simulink model "linear_sys"  (R2021b)
settings: Solver=VariableStepAuto  StartTime=0.0  StopTime=5  RelTol=1e-3
values from neighbouring files (symbols this model uses):
  beta = 15    [run_6dof.m]
  Cldp = U(21)    [totalfm.m]
  Cmdq = U(19)    [totalfm.m]
  Cmq = U(18)    [totalfm.m]
  d = 265/1000    (= 0.265)    [run_6dof.m]
  damp = 0.9    [run_6dof.m]
  g = 9.81    [run_6dof.m]
  K1 = 4.3    [run_6dof.m]
  K2 = 0.2    [run_6dof.m]
  K3 = 0.3    [run_6dof.m]
  KP = 2    [run_6dof.m]
  m = fixed_mass+N2O_mass+Fuel_mass    [CG_CPcal.m]    (also in Rocket_property.m = 168.84; totalfm.m = U(28))
  qbar = U(10)    [totalfm.m]
  S = 1/4*pi*d^2    (= 0.0551545860246)    [run_6dof.m]
  theta = acos(1-2*X/lnose)    [plotDatcomAeroGeometry_221130.m]
  tou1 = 5/wg    (= 2.5)    [run_6dof.m]
  tou2 = 1/wm*sqrt(1/afa)    [run_6dof.m]
  V = U(31)    [totalfm.m]
  wn = BW/sqrt(1-2*damp^2+sqrt(2-4*damp^2+4*damp^4))    [run_6dof.m]
undefined symbols (not defined in the file or in its folder): alpha, CAN_TRANS_FREQ, Clp, Cma, Cna, Cnq, IMU_SAMP_FREQ, Ix, Iy, n, o
libraries: simulink_extras x9, simulink x3, dspsigops x3, slctrlblks x2
settings Model: Creator=310611102  LastModifiedBy=310611102

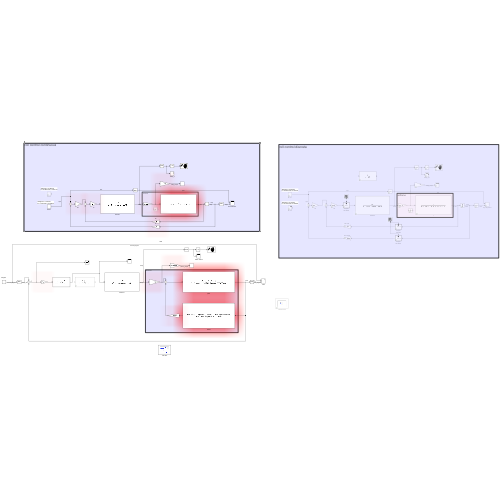
[thumbnail: Simulink's stored preview of the top-level diagram]
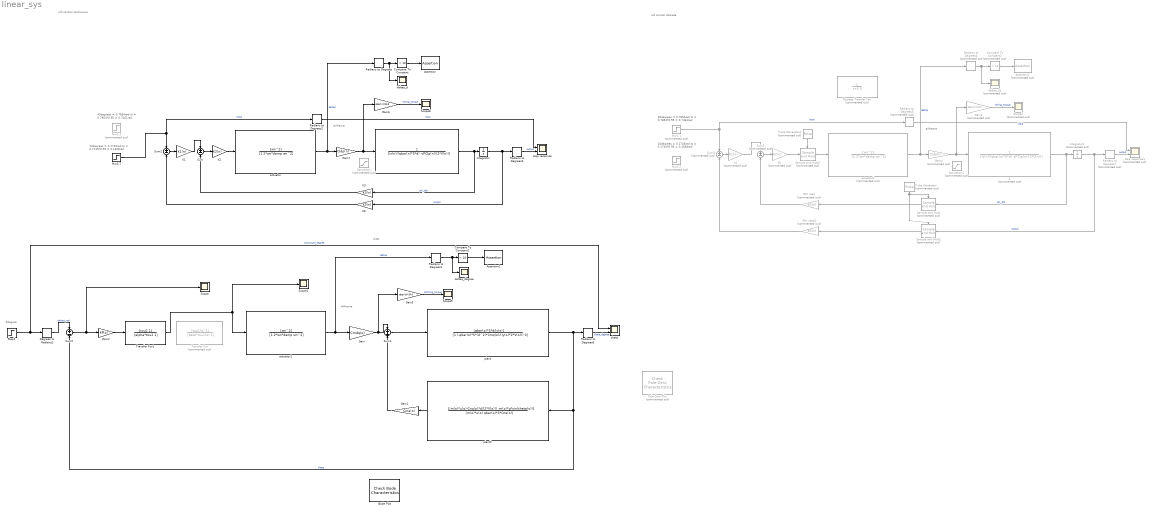
== system linear_sys ==
  note: roll control continuous
  note: 5degree
  note: airframe
  note: Airframe
  note: 45degrees = 0.7854rad
      | ts = 0.7854*0.95 = 0.7461rad
  note: C2D
  note: 10degrees = 0.1745rad
      | ts = 0.1745*0.95 = 0.1658rad
  note: airframe
  note: 45degrees = 0.7854rad
      | ts = 0.7854*0.95 = 0.7461rad
  note: 10degrees = 0.1745rad
      | ts = 0.1745*0.95 = 0.1658rad
  note: roll control discrete
  " " : TransferFcn  Numerator=1  Denominator=[Ix(n)/(qbar(n)*S*d) -d*Clp(n)/(2*V(n))]
  " 1" : TransferFcn  Commented=on  Numerator=1  Denominator=[Ix(n)/(qbar(n)*S*d) -d*Clp(n)/(2*V(n))]
  Assertion : Assertion  Enabled=off  AssertionFailFcn="error(\"large deflection angle\")"  StopWhenAssertionFail=off
  Assertion1 : Assertion  Enabled=off  AssertionFailFcn="error(\"large deflection angle\")"  StopWhenAssertionFail=off
  Assertion2 : Assertion  Commented=on  Enabled=off  AssertionFailFcn="error(\"large deflection angle\")"  StopWhenAssertionFail=off
  Bode Plot : slctrlblks/Model Verification/Check Bode  Characteristics  InstantiateOnLoad=on  SaveOperatingPoints=off  LinearizationIOs={'/Sum5', 1, 'in', 'on', '';'/plant', 1, 'out', 'on', ''}  LinearizeAt=SnapshotTimes  SnapshotTimes=[0]  TriggerType=rising  SampleTime=auto  RateConversionMethod=zoh  PreWarpFreq=10  UseExactDelayModel=off  UseFullBlockNameLabels=off  UseBusSignalLabels=off  enabled=on  stopWhenAssertionFail=off  export=off  ViewDlgPos=[1 41 1920 962]  OpenViewOnLoad=off  LaunchViewOnOpen=on  FrequencyUnits=rad/s  MagnitudeUnits=dB  PhaseUnits=deg  TimeUnits=seconds  EnableUpperBound=off  UpperBoundFrequencies=[]  UpperBoundMagnitudes=[]  EnableLowerBound=off  LowerBoundFrequencies=[]  LowerBoundMagnitudes=[]
  Compare To Constant : simulink/Logic and Bit Operations/Compare To Constant  relop=<  const=10  OutDataTypeStr=boolean
  Compare To Constant1 : simulink/Logic and Bit Operations/Compare To Constant  relop=<  const=10  OutDataTypeStr=boolean
  Compare To Constant2 : simulink/Logic and Bit Operations/Compare To Constant  Commented=on  relop=<  const=10  OutDataTypeStr=boolean
  Degrees to Radians2 : simulink_extras/Transformations/Degrees to Radians
  Discrete Transfer Fcn : DiscreteTransferFcn  Commented=on
  Gain : Gain  Gain=Cmdq(o)
  Gain1 : Gain  Gain=Cma(o)
  Gain2 : Gain  Gain=KP(o)
  Gain3 : Gain  Commented=on  Gain=qbar(n)*S*d
  Gain4 : Gain  Commented=on  Gain=Cldp(n)
  Gain5 : Gain  Gain=qbar(o)*S*d
  Gain6 : Gain  Gain=qbar(n)*S*d
  Gain7 : Gain  Gain=Cldp(n)
  IMU read : Gain  Commented=on  Gain=K3(n)
  IMU read2 : Gain  Commented=on  Gain=K3(n)
  Integrator : Integrator
  Integrator1 : Integrator  Commented=on
  K1 : Gain  Gain=K1(n)
  K2 : Gain  Gain=K2(n)
  K3 : Gain  Gain=K3(n)
  K4 : Gain  Commented=on  Gain=K1(n)
  K5 : Gain  Commented=on  Gain=K2(n)
  K6 : Gain  Gain=K3(n)
  M=0.1 : Step  Commented=on  After=45*pi/180  SampleTime=0
  M=0.2 : Step  Commented=on  After=10*pi/180  SampleTime=0
  M=0.3 : Step  Commented=on  After=45*pi/180  SampleTime=0
  M=0.7 : Step  After=10*pi/180  SampleTime=0
  Pole-Zero Plot : slctrlblks/Model Verification/Check Pole-Zero Characteristics  Commented=on  InstantiateOnLoad=on  SaveOperatingPoints=off  LinearizationIOs={'/Sum5', 1, 'in', 'on', '';'/plant', 1, 'out', 'on', ''}  LinearizeAt=SnapshotTimes  SnapshotTimes=[0]  TriggerType=rising  SampleTime=auto  RateConversionMethod=zoh  PreWarpFreq=10  UseExactDelayModel=off  UseFullBlockNameLabels=off  UseBusSignalLabels=off  enabled=on  stopWhenAssertionFail=off  export=off  ViewDlgPos=[100 200 510 390]  LaunchViewOnOpen=off  OpenViewOnLoad=off  FrequencyUnits=rad/s  MagnitudeUnits=dB  PhaseUnits=deg  TimeUnits=seconds  EnableSettlingTime=off  SettlingTime=[]  EnablePercentOvershoot=off  PercentOvershoot=[]  EnableDampingRatio=off  DampingRatio=[]  EnableNaturalFrequency=off  NaturalFrequencyBound=>=  NaturalFrequency=[]
      settings: SourceProductBaseCode=SD  SaveToWorkspace=off  SaveName=sys
  Pulse Generator : DiscretePulseGenerator  Commented=on  PulseType=Time based  Period=1/IMU_SAMP_FREQ  PulseWidth=5
  Pulse Generator1 : DiscretePulseGenerator  Commented=on  PulseType=Time based  Period=1/CAN_TRANS_FREQ  PulseWidth=5
  Radians to Degrees{,1..3,6} (5 alike) : simulink_extras/Transformations/Radians to Degrees
  Radians to Degrees4 : simulink_extras/Transformations/Radians to Degrees  Commented=on
  Radians to Degrees5 : simulink_extras/Transformations/Radians to Degrees  Commented=on
  Radians to Degrees7 : simulink_extras/Transformations/Radians to Degrees  Commented=on
  Sample and Hold : dspsigops/Sample and Hold  Commented=on  trig=Rising edge  initCond=0  latchinput=off
  Sample and Hold1 : dspsigops/Sample and Hold  Commented=on  trig=Rising edge  initCond=0  latchinput=off
  Sample and Hold2 : dspsigops/Sample and Hold  Commented=on  trig=Rising edge  initCond=0  latchinput=off
  Saturation : Saturate  Commented=on  UpperLimit=20*pi/180  LowerLimit=-20*pi/180
  Saturation1 : Saturate  Commented=on  UpperLimit=20*pi/180  LowerLimit=-20*pi/180
  Scope{,1,5..6} (4 alike) : Scope
  Scope2 : Scope  Commented=on
  Step2 : Step  After=5  SampleTime=0
  Sum : Sum  Inputs=+-
  Sum1 : Sum
  Sum2 : Sum  Inputs=+-
  Sum3 : Sum  Commented=on  Inputs=+-
  Sum4 : Sum  Commented=on  Inputs=+-
  Sum5 : Sum  Inputs=+-
  Transfer Fcn : TransferFcn  Commented=on  Numerator=[tou1(o) 1]  Denominator=[beta*tou1(o) 1]
  Transfer Fcn1 : TransferFcn  Numerator=[tou2 1]  Denominator=[alpha*tou2 1]
  actuator : TransferFcn  Numerator=[wn^2]  Denominator=[1 2*wn*damp wn^2]
  actuator1 : TransferFcn  Numerator=[wn^2]  Denominator=[1 2*wn*damp wn^2]
  actuator2 : TransferFcn  Commented=on  Numerator=[wn^2]  Denominator=[1 2*wn*damp wn^2]
  deltap_d : Scope
  deltap_d1 : Scope  Commented=on
  deltaq_degree : Scope
  plant : TransferFcn  Numerator=[qbar(o)*S*d/Iy(o)]  Denominator=[1 (-qbar(o)*S*(d^2)*Cmq(o)/(Iy(o)*2*V(o))) 0]
  plant2 : TransferFcn  Numerator=[(m(o)*u(o)-Cnq(o)*d/(2*V(o))) -m(o)*g*sin(theta(o))]  Denominator=[m(o)*u(o) qbar(o)*S*Cna(o)]
  step response : Scope  NumInputPorts=2
  step response1 : Scope  Commented=on  NumInputPorts=2
  theta : Scope  NumInputPorts=2
  wires:
  " "/1 -> K3/1, Integrator/1  "phi_dot"
  Integrator/1 -> K6/1, Radians to Degrees3/1  "output"
  actuator/1 -> Gain7/1, Radians to Degrees/1  "deltap"
  M=0.7/1 -> Radians to Degrees2/1, Sum2/1  "input"
  Radians to Degrees/1 -> deltap_d/1, Compare To Constant/1
  Compare To Constant/1 -> Assertion/1
  Sum2/1 -> K1/1
  K1/1 -> Sum/1
  K3/1 -> Sum/2
  Sum/1 -> K2/1
  Sum1/1 -> plant/1
  plant/1 -> Sum5/2, plant2/1, Radians to Degrees6/1  "theta"
  Compare To Constant1/1 -> Assertion1/1
  Radians to Degrees1/1 -> Compare To Constant1/1, deltaq_degree/1
  plant2/1 -> Gain1/1
  Gain/1 -> Gain5/1, Sum1/1
  Gain1/1 -> Sum1/2
  Radians to Degrees2/1 -> step response/1  "input"
  Radians to Degrees3/1 -> step response/2  "output"
  Radians to Degrees6/1 -> theta/2  "theta_degree"
  Step2/1 -> theta/1, Degrees to Radians2/1  "command_degree"
  Gain5/1 -> Scope5/1  "pitching_torque"
  Gain7/1 -> " "/1, Gain6/1
  Gain6/1 -> Scope6/1  "rolling_torque"
  actuator1/1 -> Radians to Degrees1/1, Gain/1  "deltaq"
  Degrees to Radians2/1 -> Sum5/1  "deltaq_rad"
  Sum5/1 -> Scope/1, Gain2/1
  Gain2/1 -> Transfer Fcn1/1
  Transfer Fcn1/1 -> actuator1/1, Scope1/1
  K2/1 -> actuator/1
  actuator2/1 -> Gain4/1, Radians to Degrees4/1  "deltap"
  " 1"/1 -> Sample and Hold/1, Integrator1/1  "phi_dot"
  K5/1 -> Sample and Hold2/1
  Gain4/1 -> " 1"/1, Gain3/1
  Gain3/1 -> Scope2/1  "rolling_torque"
  M=0.1/1 -> Sum4/1, Radians to Degrees5/1  "input"
  Compare To Constant2/1 -> Assertion2/1
  Sum4/1 -> K4/1
  IMU read/1 -> Sum3/2
  Sum3/1 -> K5/1
  K4/1 -> Sum3/1
  Radians to Degrees4/1 -> deltap_d1/1, Compare To Constant2/1
  Radians to Degrees5/1 -> step response1/1  "input"
  Radians to Degrees7/1 -> step response1/2  "output"
  Integrator1/1 -> Sample and Hold1/1, Radians to Degrees7/1  "output"
  IMU read2/1 -> Sum4/2
  Sample and Hold/1 -> IMU read/1
  Sample and Hold1/1 -> IMU read2/1
  Pulse Generator/1 -> Sample and Hold/Trigger, Sample and Hold1/Trigger
  Pulse Generator1/1 -> Sample and Hold2/Trigger
  Sample and Hold2/1 -> actuator2/1
  K6/1 -> Sum2/2
